simulink model "counter"  (R2014b)
settings: Solver=ode45  StartTime=0.0  StopTime=30.0  RelTol=1e-3
libraries: simulink x2
settings Model: Creator=kjartan  LastModifiedBy=kjartan

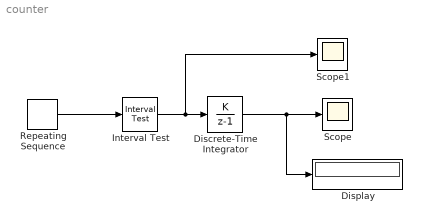
== system counter ==
  Discrete-Time Integrator : DiscreteIntegrator  IntegratorMethod=Accumulation: Forward Euler  gainval=0.001  InitialConditionSetting=State (most efficient)  SampleTime=0.001
  Display : Display
  Interval Test : simulink/Logic and Bit Operations/Interval Test  IntervalClosedRight=on  uplimit=1.2  IntervalClosedLeft=on  lowlimit=1.1  OutDataTypeStr=boolean
  Repeating Sequence : simulink/Sources/Repeating Sequence  rep_seq_t=[0, 1, 2, 3, 4]  rep_seq_y=[0 1, 2, 3, 3.5]
  Scope : Scope
      settings: YMin=0  YMax=300
  Scope1 : Scope
  wires:
  Repeating Sequence/1 -> Interval Test/1
  Interval Test/1 -> Scope1/1, Discrete-Time Integrator/1
  Discrete-Time Integrator/1 -> Display/1, Scope/1
